simulink model "rlAutoParkingValet3D"  (R2024b)
settings: Solver=VariableStepAuto  StartTime=0.0  StopTime=inf  RelTol=1e-3  AbsTol=1e-4
InitFcn:
  | if ~doTraining
  |     setupActorVehicles(mdl,freeSpotIndex);
  | end
  | egoTargetPose = parkingLot.findGoalPose(vehiclePose,freeSpotIndex,searchDist);
StartFcn:
  | if exist("visualizer","var") && ~doTraining
  |     visualizer.resetVehicle(egoInitialPose,freeSpotIndex,doTraining);
  | end
model workspace: external: MAT-File (data not in the file)
values from neighbouring files (symbols this model uses):
  centerToRear = 1.343    [autoParkingValetParams3D.m]
  doTraining = false    [RL_Parking_And_Control.m]    (also in analisis.m; lanzarSimParalelas.m)
  egoInitialPose = [40 -55 pi/2]    [RL_Parking_And_Control.m]    (also in lanzarSimParalelas.m)
  freeSpotIndex = spotsToSimulate(i)    [RL_Parking_And_Control.m]    (also in analisis.m = 18; autoParkingValetResetFcn3D.m = 21; lanzarSimParalelas.m = 18)
  info = ParkingLotManager.getInfo()    [ParkingLotManager.m]    (also in ParkingLotVisualizer.m = this.Info; RL_Parking_And_Control.m = parkingLot.getInfo(); analisis.m = parkingLot.getInfo(); autoParkingValetResetFcn3D.m)
  K_lqr = dlqr(Ad, Bd, Q, R)    [createLQRForParking3D.m]
  maxLidarDist = 20    [autoParkingValetParams3D.m]
  parkingLot = obj.ParkingLot    [ModeSelector.m]    (also in RL_Parking_And_Control.m = ParkingLotManager; analisis.m = ParkingLotManager; lanzarSimParalelas.m = ParkingLotManager)
  pTracking = 10    [createMPCForParking3D.m]    (also in createNonLinearMPCForParking3D.m)
  searchDist = 10    [RL_Parking_And_Control.m]    (also in analisis.m; lanzarSimParalelas.m)
  speedMax = 2    [autoParkingValetParams3D.m]
  steerMax = pi/4    (= 0.785398163397)    [autoParkingValetParams3D.m]
  terrTol = deg2rad(10)    [autoParkingValetParams3D.m]
  Tf = 50    [RL_Parking_And_Control.m]    (also in analisis.m; lanzarSimParalelas.m)
  trainXBounds = info.TrainingZoneXLimits    [autoParkingValetParams3D.m]    (also in autoParkingValetResetFcn3D.m = [(info.SpotLocations(freeSpotIndex,1) - 6.8125)             )
  trainYBounds = info.TrainingZoneYLimits    [autoParkingValetParams3D.m]    (also in autoParkingValetResetFcn3D.m = [(info.SpotLocations(freeSpotIndex,2) - 9.56)              ()
  Ts = 0.1    [RL_Parking_And_Control.m]    (also in analisis.m; createMPCForParking3D.m; lanzarSimParalelas.m)
  vehiclePose = [10 -32.5 pi]    [RL_Parking_And_Control.m]    (also in analisis.m; lanzarSimParalelas.m)
  xBounds = info.XLimits    [autoParkingValetParams3D.m]
  Xref = [xRef(1:p,:);repmat(xRef(end,:),Tsteps-p,1)]    [ParkingLotManager.m]    (also in createLQRForParking3D.m = parkingLot.createReferenceTrajectory(Ts, Tf); createMPCForParking3D.m = ParkingLotManager.createReferenceTrajectory(Ts,Tf); createNonLinearMPCForParking3D.m = ParkingLotManager.createReferenceTrajectory(Ts,Tf))
  xyerrTol = 0.75    [autoParkingValetParams3D.m]
  yBounds = info.YLimits    [autoParkingValetParams3D.m]
undefined symbols (not defined in the file or in its folder): Sim3dSensor
libraries: sim3dautolib x23, simulink_extras x23, mpclib x2, rllib x1, robotmobilelib x1, sim3dphyssensorlib x1, sim3dlib x1
(part 1 of 2)
settings Model: PauseTimes=24.5  PacingRate=0.089000  Creator=The MathWorks, Inc.  LastModifiedBy=josea
settings SolverCC: AutoScaleAbsTol=off  AlgebraicLoopSolver=TrustRegion  MinimalZcImpactIntegration=on  MaxZcPerStep=1
settings DataIOCC: SaveOutput=off  DSMLogging=off  SaveTime=off
settings DebuggingCC: UnconnectedInputMsg=warning  UnconnectedOutputMsg=warning  UnconnectedLineMsg=warning
settings ModelReferenceCC: EnableRefExpFcnMdlSchedulingChecks=on
settings RTWCC: GPUComputeCapability=3.5  DLArmComputeVersion=19.05

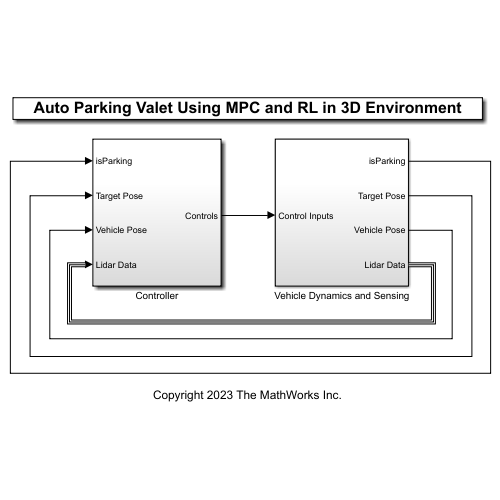
[thumbnail: Simulink's stored preview of the top-level diagram]
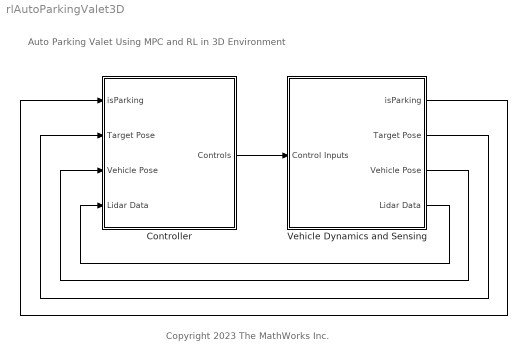
== system rlAutoParkingValet3D ==
  note: Copyright 2023 The MathWorks Inc.
  note: Auto Parking Valet Using MPC and RL in 3D Environment
  Controller : Subsystem
  Vehicle Dynamics and Sensing : Subsystem
  wires:
  Controller/1(Controls) -> Vehicle Dynamics and Sensing/1(Control Inputs)
  Vehicle Dynamics and Sensing/1(isParking) -> Controller/1(isParking)
  Vehicle Dynamics and Sensing/2(Target Pose) -> Controller/2(Target Pose)
  Vehicle Dynamics and Sensing/3(Vehicle Pose) -> Controller/3(Vehicle Pose)
  Vehicle Dynamics and Sensing/4(Lidar Data) -> Controller/4(Lidar Data)

== system rlAutoParkingValet3D/Controller ==
  isParking : Inport
  Target Pose : Inport  Port=2
  Vehicle Pose : Inport  Port=3
  Lidar Data : Inport  Port=4
  MPC Tracking Controller : Subsystem
  Merge : Merge
  NOT : Logic  Operator=NOT  AllPortsSameDT=off  OutDataTypeStr=boolean
  RL Controller : Subsystem
  Controls : Outport
  wires:
  Merge/1 -> Controls/1
  Vehicle Pose/1 -> RL Controller/2(Vehicle Pose), MPC Tracking Controller/1(States)
  Target Pose/1 -> RL Controller/1(Target Pose)
  Lidar Data/1 -> RL Controller/3(Lidar Data)
  RL Controller/1(Controls) -> Merge/2
  MPC Tracking Controller/1(Controls) -> Merge/1
  isParking/1 -> NOT/1, RL Controller/Enable
  NOT/1 -> MPC Tracking Controller/Enable

== system rlAutoParkingValet3D/Vehicle Dynamics and Sensing ==
  Control Inputs : Inport
  Demux : Demux  Outputs=2
  Ego Vehicle Model : Subsystem
  Unreal Engine Visualization and Sensing : Subsystem  InitFcn=|  VariantControl=UnrealOn  mask{EnableUEViz=on, EnablePCViz=on}
      | enableUEViz = get_param(gcb,'enableUEViz');
      | enablePCPlayer = get_param(gcb,'enablePCViz');
      | sim3DConfigBlock = strcat(gcb, "/Simulation 3D Scene Configuration");
      | pcViewerBlock = strcat(gcb, "/Point Cloud Viewer");
      | 
      | if strcmp(enableUEViz, "on")
      |     set_param(sim3DConfigBlock, "EnableWindow", "on");
      | elseif strcmp(enableUEViz, "off")
      |     set_param(sim3DConfigBlock, "EnableWindow", "off");
      | end
      | 
      | if strcmp(enablePCPlayer, "on")
      |     set_param(pcViewerBlock, "OpenAtMdlStart", "on");
      | elseif strcmp(enablePCPlayer, "off")
      |     set_param(pcViewerBlock, "OpenAtMdlStart", "off");
      | end
      mask prompts: EnableUEViz "Enable Unreal Engine visualization"; EnablePCViz "Enable point cloud visualization"
      mask init:
      | enableUEViz = EnableUEViz;
      | enablePCViz = EnablePCViz;
  Vehicle Mode Selector : Subsystem
  isParking : Outport
  Target Pose : Outport  Port=2
  Vehicle Pose : Outport  Port=3
  Lidar Data : Outport  Port=4
  wires:
  Ego Vehicle Model/1(Vehicle Pose (Centroid)) -> Unreal Engine Visualization and Sensing/2(Vehicle Pose (Center)), Vehicle Mode Selector/1(Vehicle Pose)
  Demux/2 -> Unreal Engine Visualization and Sensing/4(Steer Angle), Ego Vehicle Model/2(Steering (rad))  "steering"
  Demux/1 -> Ego Vehicle Model/1(Speed (m/s))
  Unreal Engine Visualization and Sensing/1(Lidar Data) -> Lidar Data/1
  Control Inputs/1 -> Demux/1
  Vehicle Mode Selector/2(isParking) -> isParking/1, Unreal Engine Visualization and Sensing/1(isParking)  "isParking"
  Vehicle Mode Selector/1(TargetPose) -> Target Pose/1
  Ego Vehicle Model/2(Vehicle Pose (Rear Axle)) -> Vehicle Pose/1, Unreal Engine Visualization and Sensing/3(Vehicle Pose (Rear Axle))  "egoPose"

== system rlAutoParkingValet3D/Controller/MPC Tracking Controller ==
  States : Inport
  Enable : EnablePort  StatesWhenEnabling=reset
  Variant Subsystem : Subsystem  Variant=on  VariantControlMode=label  LabelModeActiveChoice=Choice_3  mask{choice=Pure Pursuit}
      mask init:
      | choice = get_param(gcb,'choice');
      | vssBlk = gcb;
      | oldVariant = get_param(gcb,'LabelModeActiveChoice');
      | if strcmp(choice,'Adaptive MPC')
      |     
      |     set_param(vssBlk, 'LabelModeActiveChoice', 'Choice_1');
      | elseif strcmp(choice,'LQR')
      |     
      |     set_param(vssBlk, 'LabelModeActiveChoice', 'Choice_2');
      | elseif strcmp(choice,'Pure Pursuit')
      |     
      |     set_param(vssBlk, 'LabelModeActiveChoice', 'Choice_3');
      | elseif strcmp(choice,'Stanley')
      |     
      |     set_param(vssBlk, 'LabelModeActiveChoice', 'Choice_4');
      | elseif strcmp(choice,'Nonlinear MPC')
      |     
      |     set_param(vssBlk, 'LabelModeActiveChoice', 'Choice_5');
      | end
      mask TypeOptions choice: Adaptive MPC | LQR | Pure Pursuit | Stanley | Nonlinear MPC
  Controls : Outport
  wires:
  States/1 -> Variant Subsystem/1(states)
  Variant Subsystem/1(controls) -> Controls/1

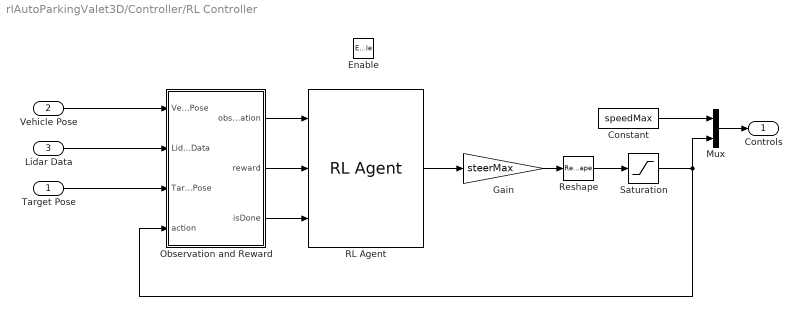
== system rlAutoParkingValet3D/Controller/RL Controller ==
  Target Pose : Inport
  Vehicle Pose : Inport  Port=2
  Lidar Data : Inport  Port=3
  Enable : EnablePort  StatesWhenEnabling=reset
  Constant : Constant  Value=speedMax
  Gain : Gain  Gain=steerMax
  Mux : Mux  Inputs=2
  Observation and Reward : Subsystem
  RL Agent : rllib/RL Agent  Agent=agent  ExternalActionAsInput=off  ProvideLastAction=off  ProvideCumRwd=off  TreatAsDirectFeedthrough=on  UseStrictObservationDataTypes=off
  Reshape : Reshape
  Saturation : Saturate  UpperLimit=steerMax  LowerLimit=-steerMax
  Controls : Outport
  wires:
  Observation and Reward/1(observation) -> RL Agent/1
  Observation and Reward/2(reward) -> RL Agent/2
  Vehicle Pose/1 -> Observation and Reward/1(Vehicle Pose)
  Target Pose/1 -> Observation and Reward/3(Target Pose)
  RL Agent/1 -> Gain/1
  Saturation/1 -> Mux/2, Observation and Reward/4(action)
  Reshape/1 -> Saturation/1
  Constant/1 -> Mux/1
  Mux/1 -> Controls/1
  Gain/1 -> Reshape/1
  Observation and Reward/3(isDone) -> RL Agent/3
  Lidar Data/1 -> Observation and Reward/2(Lidar Data)

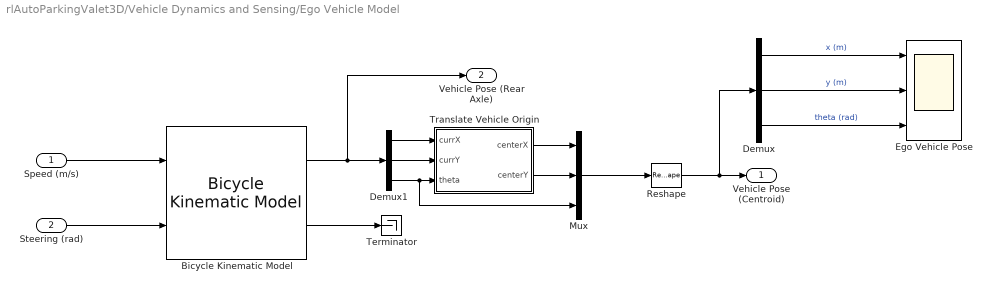
== system rlAutoParkingValet3D/Vehicle Dynamics and Sensing/Ego Vehicle Model ==
  Speed (m/s) : Inport
  Steering (rad) : Inport  Port=2
  Bicycle Kinematic Model : robotmobilelib/Bicycle Kinematic Model  VehicleInputs=Vehicle Speed & Steering Angle  WheelBase=info.CenterToRearDist+info.CenterToFrontDist  VehicleSpeedRange=[-5, 5]  MaxSteeringAngle=steerMax  InitialState=egoInitialPose  SimulateUsing=Interpreted execution
  Demux : Demux  Outputs=3
  Demux1 : Demux  Outputs=3
  Ego Vehicle Pose : Scope  NumInputPorts=3
  Mux : Mux  Inputs=3
  Reshape : Reshape
  Terminator : Terminator
  Translate Vehicle Origin : Subsystem
  Vehicle Pose (Centroid) : Outport
  Vehicle Pose (Rear Axle) : Outport  Port=2
  wires:
  Demux/3 -> Ego Vehicle Pose/3  "theta (rad)"
  Demux/1 -> Ego Vehicle Pose/1  "x (m)"
  Demux/2 -> Ego Vehicle Pose/2  "y (m)"
  Speed (m/s)/1 -> Bicycle Kinematic Model/1
  Steering (rad)/1 -> Bicycle Kinematic Model/2
  Mux/1 -> Reshape/1
  Bicycle Kinematic Model/2 -> Terminator/1
  Bicycle Kinematic Model/1 -> Demux1/1, Vehicle Pose (Rear Axle)/1
  Reshape/1 -> Demux/1, Vehicle Pose (Centroid)/1
  Translate Vehicle Origin/2(centerY) -> Mux/2
  Demux1/1 -> Translate Vehicle Origin/1(currX)
  Demux1/3 -> Mux/3, Translate Vehicle Origin/3(theta)
  Translate Vehicle Origin/1(centerX) -> Mux/1
  Demux1/2 -> Translate Vehicle Origin/2(currY)

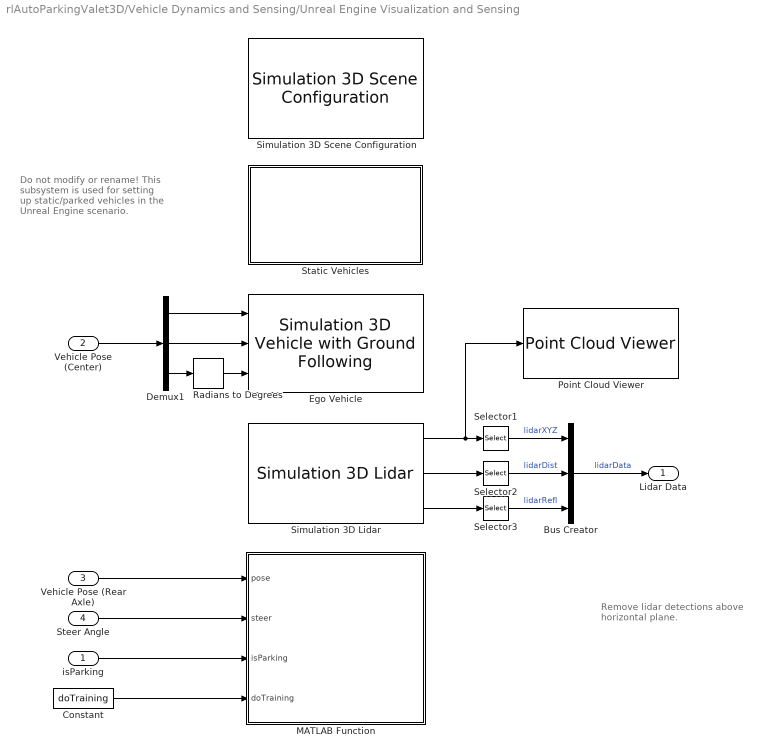
== system rlAutoParkingValet3D/Vehicle Dynamics and Sensing/Unreal Engine Visualization and Sensing ==
  note: Remove lidar detections above horizontal plane.
  note: Do not modify or rename!
      |
      | This subsystem is used for setting up static/parked vehicles in the Unreal Engine scenario.
  isParking : Inport
  Vehicle Pose (Center) : Inport  Port=2
  Vehicle Pose (Rear Axle) : Inport  Port=3
  Steer Angle : Inport  Port=4
  Bus Creator : BusCreator  Inputs=3
  Constant : Constant  Value=doTraining
  Demux1 : Demux  Outputs=3
  Ego Vehicle : sim3dautolib/Simulation 3D Vehicle with Ground Following  Priority=-1  PassVehMesh=Hatchback  MeshPath=/MathWorksSimulation/Vehicles/Muscle/Meshes/SK_MuscleCar.SK_MuscleCar  TrackWidth=1.9  WheelBase=3  WheelRadius=0.35  VehColor=Red  InitialPos=[egoInitialPose(1)+cos(egoInitialPose(3))*centerToRear, egoInitialPose(2)+sin(egoInitialPose(3))*centerToRear, 0]  InitialRot=[0, 0, rad2deg(egoInitialPose(3))]  ActorName=EgoVehicle  SampleTime=-1  ActorType=SimulinkVehicle  ID=C  aMode=3  ActorTag=EgoVehicle  CoordinateScheme=ISO  VehLightsControl=off  HeadlightColor=[ 1, 1, 1 ]  HighBeamIntensity=100000  LowBeamIntensity=60000  HighBeamConeAngle=70  LowBeamConeAngle=70  LeftHeadlightOrientation=[ 0, 0 ]  RightHeadlightOrientation=[ 0, 0 ]  BrakelightIntensity=500  ReverselightIntensity=500  SignallightIntensity=500  SignallightPeriod=1  SignalPulseWidth=50  TransformOutportEnabled=off
      settings: LibrarySourceBlock=drivingsim3d/Simulation 3D Vehicle with Ground Following
  MATLAB Function : MATLAB Function  TreatAsAtomicUnit=on
  Point Cloud Viewer : PointCloudViewer  FigPos=[857.8 630 539.2 508.8]
  Radians to Degrees : simulink_extras/Transformations/Radians to Degrees
  Selector1 : Selector  NumberOfDimensions=3  InputPortWidth=3  IndexOptions=Index vector (dialog),Select all,Select all  Indices=45:60,1,1  OutputSizes=1,1,1
  Selector2 : Selector  NumberOfDimensions=2  InputPortWidth=3  IndexOptions=Index vector (dialog),Select all  Indices=45:60,1  OutputSizes=1,1
  Selector3 : Selector  NumberOfDimensions=2  InputPortWidth=3  IndexOptions=Index vector (dialog),Select all  Indices=45:60,1  OutputSizes=1,1
  Simulation 3D Lidar : sim3dphyssensorlib/Simulation 3D Lidar  Priority=1  sensorTag=Sim3dSensor�  sensorId=2  sensorName=Sim3dSensor�  vehTagList={'EgoVehicle';'Scene Origin';'Vehicle1';'Vehicle10';'Vehicle11';'Vehicle12';'Vehicle13';'Vehicle14';'Vehicle15';'Vehicle16';'Vehicle17';'Vehicle18';'Vehicle19';'Vehicle2';'Vehicle20';'Vehicle21';'Vehicle22';'Vehicle23';'Vehicle3';'Vehicle4';'Vehicle5';'Vehicle6';'Vehicle7';'Vehicle9'}  vehTag=EgoVehicle  mountLoc=Roof center  offsetFlag=on  tmountOffset=[0, 0, 0.2]  rmountOffset=[0, 0, 0]  DetectionRange=maxLidarDist  RangeResolution=0.002  VerticalFOV=lidarVerticalFOV  VerticalResolution=lidarVerticalRes  HorizontalFOV=lidarHorizontalFOV  HorizontalResolution=lidarHorizontalRes  DistanceOutportEnabled=on  ReflectivityOutportEnabled=on  SemanticOutportEnabled=off  TransformOutportEnabled=off  SampleTime=-1  mountPoint=[0 0 1.76]  mountOrientation=[0 0 0]  aMode=3  ID=2
      settings: LibrarySourceBlock=drivingsim3d/Simulation 3D Lidar
  Simulation 3D Scene Configuration : sim3dlib/Simulation 3D Scene Configuration  Priority=0  ProjectFormat=Default Scenes  SceneDesc=Large parking lot  ProjectName=C:\Program Files\MATLAB\R2024b\toolbox\shared\sim3d_projects\automotive_project_windows\UE\WindowsNoEditor\VehicleSimulation.exe  ScenePath=/Game/Maps/HwStrght  EnableOpenDRIVE=off  vehTagList={'Custom';'EgoVehicle';'Scene Origin';'Vehicle1';'Vehicle10';'Vehicle11';'Vehicle12';'Vehicle13';'Vehicle14';'Vehicle15';'Vehicle16';'Vehicle17';'Vehicle18';'Vehicle19';'Vehicle2';'Vehicle20';'Vehicle21';'Vehicle22';'Vehicle23';'Vehicle3';'Vehicle4';'Vehicle5';'Vehicle6';'Vehicle7';'Vehicle9'}  vehTag=EgoVehicle  FreeCameraInitialTranslation=[0, 0, 0]  FreeCameraDefaultInitialTranslation=[-6, 0, 2]  FreeCameraInitialRotation=[0, 0, 0]  FreeCameraDefaultInitialRotation=[0, -15, 0]  OpVisEn=off  Ts=Ts  EnableWindow=on  EnableRemoteAccess=off  EnableWeather=off  SunAzimuth=90  SunAltitude=40.0  EnableGeospatialSun=off  Latitude=0  Longitude=0  Date=2023-01-01  Time=10:30:00  GeoTimeZone=-5.0  SunDaylightSaving=off  wind=1  clouds=10  EnableVolumetricClouds=off  CloudCoverage=0  CloudAltitude=6  fog=0  rain=0  RaindropsEffect=off  SnowDensity=0  EnableGeospatial=off  UseTrueOrigin=off  OriginHeight=200  OriginLatitude=40.744652  OriginLongitude=-73.988864  MapStyle=Aerial  AdditionalAssetIDs=[]  UseAdvancedSunSky=off  SolarTime=11  TimeZone=-5  Day=21  Month=9  Year=2022  UseDaylightSavingTime=on  DSTStartDay=10  DSTStartMonth=3  DSTEndDay=3  DSTEndMonth=11  DSTSwitchHour=2  sensorTag=MainCamera2  sensorId=2  sensorName=MainCamera2  mountLoc=Origin  offsetFlag=off  tmountOffset=[0, 0, 0]  rmountOffset=[0, 0, 0]  HorizontalResolution=1280  VerticalResolution=720  HorizontalFOV=60  mountPoint=[0 0 0]  mountOrientation=[0 0 0]  aMode=3  ID=2  GeoTrigger=Inactive
      settings: LibrarySourceBlock=drivingsim3d/Simulation 3D Scene Configuration
  Static Vehicles : Subsystem  Priority=-1
  Lidar Data : Outport
  wires:
  Vehicle Pose (Center)/1 -> Demux1/1
  Radians to Degrees/1 -> Ego Vehicle/3
  Demux1/1 -> Ego Vehicle/1
  Demux1/2 -> Ego Vehicle/2
  Demux1/3 -> Radians to Degrees/1
  Simulation 3D Lidar/1 -> Point Cloud Viewer/1, Selector1/1
  Simulation 3D Lidar/2 -> Selector2/1
  Simulation 3D Lidar/3 -> Selector3/1
  Bus Creator/1 -> Lidar Data/1  "lidarData"
  Selector1/1 -> Bus Creator/1  "lidarXYZ"
  Selector2/1 -> Bus Creator/2  "lidarDist"
  Selector3/1 -> Bus Creator/3  "lidarRefl"
  Steer Angle/1 -> MATLAB Function/2(steer)
  isParking/1 -> MATLAB Function/3(isParking)
  Constant/1 -> MATLAB Function/4(doTraining)
  Vehicle Pose (Rear Axle)/1 -> MATLAB Function/1(pose)

== system rlAutoParkingValet3D/Vehicle Dynamics and Sensing/Vehicle Mode Selector ==
  Vehicle Pose : Inport
  Constant : Constant  Value=doTraining
  Constant1 : Constant  Value=egoTargetPose
  Hold : Subsystem
  Mode Selector : MATLABSystem  System=ModeSelector  MaxDepth=searchDist  MaxViewAngle=2*pi/3  FreeSpotIndex=freeSpotIndex  ParkingLot=parkingLot
      mask Type: ModeSelector
      mask Display:
      | disp(['Mode' char(10) 'Selector']);
      | port_label('input',1,'Ego Pose');
      | port_label('output',1,'Spot Found');
      | port_label('output',2,'Target Spot Pose');
  OR : Logic  Operator=OR  AllPortsSameDT=off  OutDataTypeStr=boolean
  Switch : Switch  Threshold=1  SaturateOnIntegerOverflow=off  InputSameDT=off
  TargetPose : Outport
  isParking : Outport  Port=2
  wires:
  Hold/1(y) -> isParking/1
  Switch/1 -> TargetPose/1
  Vehicle Pose/1 -> Mode Selector/1
  Mode Selector/2 -> Switch/3
  Constant/1 -> Switch/2, OR/2
  Constant1/1 -> Switch/1
  OR/1 -> Hold/1(u)
  Mode Selector/1 -> OR/1

== system rlAutoParkingValet3D/Controller/MPC Tracking Controller/Variant Subsystem ==
  note: 1) Add Subsystem or Model blocks as valid variant choices.
      | 2) You cannot connect blocks at this level. At simulation, connectivity is automatically
      | determined, based on the active variant and port name matching.
  states : Inport
  Adaptive MPC : Subsystem  VariantControl=Choice_1
  LQR : Subsystem  VariantControl=Choice_2
  Nonlinear MPC : Subsystem  VariantControl=Choice_5
  Pure Pursuit : Subsystem  VariantControl=Choice_3
  Stanley : Subsystem  VariantControl=Choice_4
  controls : Outport

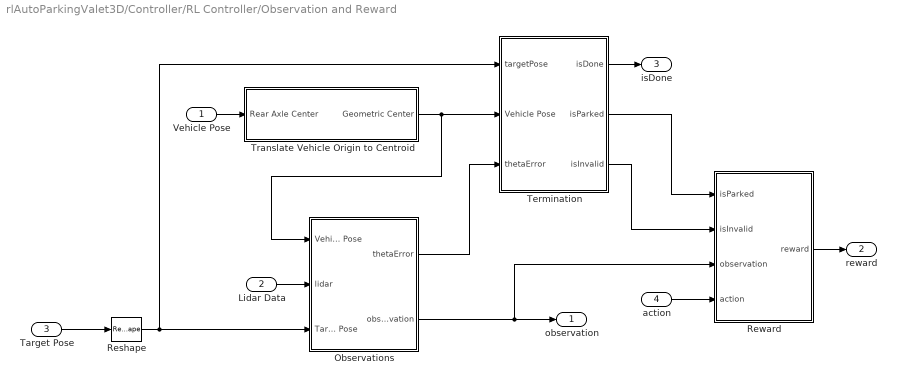
== system rlAutoParkingValet3D/Controller/RL Controller/Observation and Reward ==
  Vehicle Pose : Inport
  Lidar Data : Inport  Port=2
  Target Pose : Inport  Port=3
  action : Inport  Port=4
  Observations : Subsystem
  Reshape : Reshape
  Reward : Subsystem
  Termination : Subsystem
  Translate Vehicle Origin to Centroid : Subsystem
  observation : Outport
  reward : Outport  Port=2
  isDone : Outport  Port=3
  wires:
  action/1 -> Reward/4(action)
  Reward/1(reward) -> reward/1
  Target Pose/1 -> Reshape/1
  Observations/2(observation) -> observation/1, Reward/3(observation)
  Lidar Data/1 -> Observations/2(lidar)
  Termination/2(isParked) -> Reward/1(isParked)
  Reshape/1 -> Observations/3(Target Pose), Termination/1(targetPose)
  Termination/1(isDone) -> isDone/1
  Termination/3(isInvalid) -> Reward/2(isInvalid)
  Translate Vehicle Origin to Centroid/1(Geometric Center) -> Observations/1(Vehicle Pose), Termination/2(Vehicle Pose)
  Vehicle Pose/1 -> Translate Vehicle Origin to Centroid/1(Rear Axle Center)
  Observations/1(thetaError) -> Termination/3(thetaError)

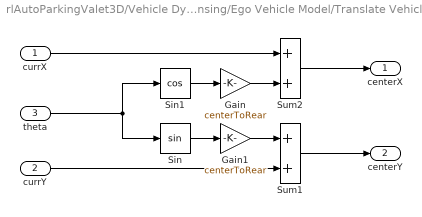
== system rlAutoParkingValet3D/Vehicle Dynamics and Sensing/Ego Vehicle Model/Translate Vehicle Origin ==
  currX : Inport
  currY : Inport  Port=2
  theta : Inport  Port=3
  Gain : Gain  Gain=centerToRear
  Gain1 : Gain  Gain=centerToRear
  Sin : Trigonometry
  Sin1 : Trigonometry  Operator=cos
  Sum1 : Sum
  Sum2 : Sum
  centerX : Outport
  centerY : Outport  Port=2
  wires:
  Sum1/1 -> centerY/1
  currY/1 -> Sum1/2
  theta/1 -> Sin/1, Sin1/1
  Sin/1 -> Gain1/1
  Sin1/1 -> Gain/1
  currX/1 -> Sum2/1
  Sum2/1 -> centerX/1
  Gain/1 -> Sum2/2
  Gain1/1 -> Sum1/1

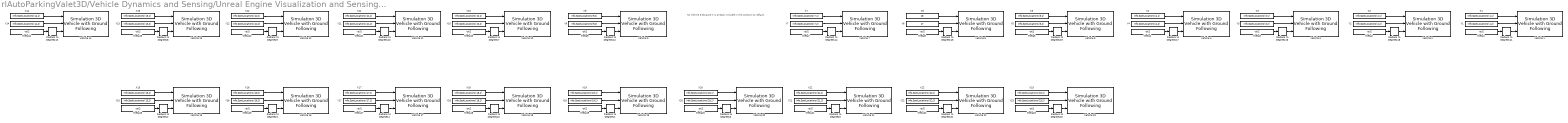
== system rlAutoParkingValet3D/Vehicle Dynamics and Sensing/Unreal Engine Visualization and Sensing/Static Vehicles ==
  note: No Vehicle 8 because it is already included in the scenario by default.
  Radians to Degrees{1..22} (22 alike) : simulink_extras/Transformations/Radians to Degrees
  Vehicle 1 : sim3dautolib/Simulation 3D Vehicle with Ground Following  Priority=-1  PassVehMesh=Sedan  MeshPath=/MathWorksAutomotiveContent/Vehicles/Muscle/Meshes/SK_MuscleCar.SK_MuscleCar  TrackWidth=1.9  WheelBase=3  WheelRadius=0.35  VehColor=White  InitialPos=[info.SpotLocations(1,1), info.SpotLocations(1,2), 0]  InitialRot=[0 0 -pi/2]  ActorName=Vehicle1  SampleTime=Ts  ActorType=SimulinkVehicle  ID=C  aMode=3  ActorTag=Vehicle1  CoordinateScheme=ISO  VehLightsControl=off  HeadlightColor=[ 1, 1, 1 ]  HighBeamIntensity=100000  LowBeamIntensity=60000  HighBeamConeAngle=70  LowBeamConeAngle=70  LeftHeadlightOrientation=[ 0, 0 ]  RightHeadlightOrientation=[ 0, 0 ]  BrakelightIntensity=500  ReverselightIntensity=500  SignallightIntensity=500  SignallightPeriod=1  SignalPulseWidth=50  TransformOutportEnabled=off
      settings: LibrarySourceBlock=drivingsim3d/Simulation 3D Vehicle with Ground Following
  Vehicle 10 : sim3dautolib/Simulation 3D Vehicle with Ground Following  Priority=-1  PassVehMesh=Sedan  MeshPath=/MathWorksAutomotiveContent/Vehicles/Muscle/Meshes/SK_MuscleCar.SK_MuscleCar  TrackWidth=1.9  WheelBase=3  WheelRadius=0.35  VehColor=Red  InitialPos=[info.SpotLocations(10,1), info.SpotLocations(10,2), 0]  InitialRot=[0 0 -pi/2]  ActorName=Vehicle10  SampleTime=Ts  ActorType=SimulinkVehicle  ID=C  aMode=3  ActorTag=Vehicle10  CoordinateScheme=ISO  VehLightsControl=off  HeadlightColor=[ 1, 1, 1 ]  HighBeamIntensity=100000  LowBeamIntensity=60000  HighBeamConeAngle=70  LowBeamConeAngle=70  LeftHeadlightOrientation=[ 0, 0 ]  RightHeadlightOrientation=[ 0, 0 ]  BrakelightIntensity=500  ReverselightIntensity=500  SignallightIntensity=500  SignallightPeriod=1  SignalPulseWidth=50  TransformOutportEnabled=off
      settings: LibrarySourceBlock=drivingsim3d/Simulation 3D Vehicle with Ground Following
  Vehicle 11 : sim3dautolib/Simulation 3D Vehicle with Ground Following  Priority=-1  PassVehMesh=Muscle car  MeshPath=/MathWorksAutomotiveContent/Vehicles/Muscle/Meshes/SK_MuscleCar.SK_MuscleCar  TrackWidth=1.9  WheelBase=3  WheelRadius=0.35  VehColor=Black  InitialPos=[info.SpotLocations(11,1), info.SpotLocations(11,2), 0]  InitialRot=[0 0 -pi/2]  ActorName=Vehicle11  SampleTime=Ts  ActorType=SimulinkVehicle  ID=C  aMode=3  ActorTag=Vehicle11  CoordinateScheme=ISO  VehLightsControl=off  HeadlightColor=[ 1, 1, 1 ]  HighBeamIntensity=100000  LowBeamIntensity=60000  HighBeamConeAngle=70  LowBeamConeAngle=70  LeftHeadlightOrientation=[ 0, 0 ]  RightHeadlightOrientation=[ 0, 0 ]  BrakelightIntensity=500  ReverselightIntensity=500  SignallightIntensity=500  SignallightPeriod=1  SignalPulseWidth=50  TransformOutportEnabled=off
      settings: LibrarySourceBlock=drivingsim3d/Simulation 3D Vehicle with Ground Following
  Vehicle 12 : sim3dautolib/Simulation 3D Vehicle with Ground Following  Priority=-1  PassVehMesh=Sport utility vehicle  MeshPath=/MathWorksAutomotiveContent/Vehicles/Muscle/Meshes/SK_MuscleCar.SK_MuscleCar  TrackWidth=1.9  WheelBase=3  WheelRadius=0.35  VehColor=White  InitialPos=[info.SpotLocations(12,1), info.SpotLocations(12,2), 0]  InitialRot=[0 0 -pi/2]  ActorName=Vehicle12  SampleTime=Ts  ActorType=SimulinkVehicle  ID=C  aMode=3  ActorTag=Vehicle12  CoordinateScheme=ISO  VehLightsControl=off  HeadlightColor=[ 1, 1, 1 ]  HighBeamIntensity=100000  LowBeamIntensity=60000  HighBeamConeAngle=70  LowBeamConeAngle=70  LeftHeadlightOrientation=[ 0, 0 ]  RightHeadlightOrientation=[ 0, 0 ]  BrakelightIntensity=500  ReverselightIntensity=500  SignallightIntensity=500  SignallightPeriod=1  SignalPulseWidth=50  TransformOutportEnabled=off
      settings: LibrarySourceBlock=drivingsim3d/Simulation 3D Vehicle with Ground Following
  Vehicle 13 : sim3dautolib/Simulation 3D Vehicle with Ground Following  Priority=-1  PassVehMesh=Sedan  MeshPath=/MathWorksAutomotiveContent/Vehicles/Muscle/Meshes/SK_MuscleCar.SK_MuscleCar  TrackWidth=1.9  WheelBase=3  WheelRadius=0.35  VehColor=Blue  InitialPos=[info.SpotLocations(13,1), info.SpotLocations(13,2), 0]  InitialRot=[0 0 -pi/2]  ActorName=Vehicle13  SampleTime=Ts  ActorType=SimulinkVehicle  ID=C  aMode=3  ActorTag=Vehicle13  CoordinateScheme=ISO  VehLightsControl=off  HeadlightColor=[ 1, 1, 1 ]  HighBeamIntensity=100000  LowBeamIntensity=60000  HighBeamConeAngle=70  LowBeamConeAngle=70  LeftHeadlightOrientation=[ 0, 0 ]  RightHeadlightOrientation=[ 0, 0 ]  BrakelightIntensity=500  ReverselightIntensity=500  SignallightIntensity=500  SignallightPeriod=1  SignalPulseWidth=50  TransformOutportEnabled=off
      settings: LibrarySourceBlock=drivingsim3d/Simulation 3D Vehicle with Ground Following
  Vehicle 14 : sim3dautolib/Simulation 3D Vehicle with Ground Following  Priority=-1  PassVehMesh=Sedan  MeshPath=/MathWorksAutomotiveContent/Vehicles/Muscle/Meshes/SK_MuscleCar.SK_MuscleCar  TrackWidth=1.9  WheelBase=3  WheelRadius=0.35  VehColor=Blue  InitialPos=[info.SpotLocations(14,1), info.SpotLocations(14,2), 0]  InitialRot=[0 0 -pi/2]  ActorName=Vehicle14  SampleTime=Ts  ActorType=SimulinkVehicle  ID=C  aMode=3  ActorTag=Vehicle14  CoordinateScheme=ISO  VehLightsControl=off  HeadlightColor=[ 1, 1, 1 ]  HighBeamIntensity=100000  LowBeamIntensity=60000  HighBeamConeAngle=70  LowBeamConeAngle=70  LeftHeadlightOrientation=[ 0, 0 ]  RightHeadlightOrientation=[ 0, 0 ]  BrakelightIntensity=500  ReverselightIntensity=500  SignallightIntensity=500  SignallightPeriod=1  SignalPulseWidth=50  TransformOutportEnabled=off
      settings: LibrarySourceBlock=drivingsim3d/Simulation 3D Vehicle with Ground Following
  Vehicle 15 : sim3dautolib/Simulation 3D Vehicle with Ground Following  Priority=-1  PassVehMesh=Sedan  MeshPath=/MathWorksAutomotiveContent/Vehicles/Muscle/Meshes/SK_MuscleCar.SK_MuscleCar  TrackWidth=1.9  WheelBase=3  WheelRadius=0.35  VehColor=Blue  InitialPos=[info.SpotLocations(15,1), info.SpotLocations(15,2), 0]  InitialRot=[0 0 -pi/2]  ActorName=Vehicle15  SampleTime=Ts  ActorType=SimulinkVehicle  ID=C  aMode=3  ActorTag=Vehicle15  CoordinateScheme=ISO  VehLightsControl=off  HeadlightColor=[ 1, 1, 1 ]  HighBeamIntensity=100000  LowBeamIntensity=60000  HighBeamConeAngle=70  LowBeamConeAngle=70  LeftHeadlightOrientation=[ 0, 0 ]  RightHeadlightOrientation=[ 0, 0 ]  BrakelightIntensity=500  ReverselightIntensity=500  SignallightIntensity=500  SignallightPeriod=1  SignalPulseWidth=50  TransformOutportEnabled=off
      settings: LibrarySourceBlock=drivingsim3d/Simulation 3D Vehicle with Ground Following
  Vehicle 16 : sim3dautolib/Simulation 3D Vehicle with Ground Following  Priority=-1  PassVehMesh=Sport utility vehicle  MeshPath=/MathWorksAutomotiveContent/Vehicles/Muscle/Meshes/SK_MuscleCar.SK_MuscleCar  TrackWidth=1.9  WheelBase=3  WheelRadius=0.35  VehColor=White  InitialPos=[info.SpotLocations(16,1), info.SpotLocations(16,2), 0]  InitialRot=[0 0 -pi/2]  ActorName=Vehicle16  SampleTime=Ts  ActorType=SimulinkVehicle  ID=C  aMode=3  ActorTag=Vehicle16  CoordinateScheme=ISO  VehLightsControl=off  HeadlightColor=[ 1, 1, 1 ]  HighBeamIntensity=100000  LowBeamIntensity=60000  HighBeamConeAngle=70  LowBeamConeAngle=70  LeftHeadlightOrientation=[ 0, 0 ]  RightHeadlightOrientation=[ 0, 0 ]  BrakelightIntensity=500  ReverselightIntensity=500  SignallightIntensity=500  SignallightPeriod=1  SignalPulseWidth=50  TransformOutportEnabled=off
      settings: LibrarySourceBlock=drivingsim3d/Simulation 3D Vehicle with Ground Following
  Vehicle 17 : sim3dautolib/Simulation 3D Vehicle with Ground Following  Priority=-1  PassVehMesh=Hatchback  MeshPath=/MathWorksAutomotiveContent/Vehicles/Muscle/Meshes/SK_MuscleCar.SK_MuscleCar  TrackWidth=1.9  WheelBase=3  WheelRadius=0.35  VehColor=Blue  InitialPos=[info.SpotLocations(17,1), info.SpotLocations(17,2), 0]  InitialRot=[0 0 -pi/2]  ActorName=Vehicle17  SampleTime=Ts  ActorType=SimulinkVehicle  ID=C  aMode=3  ActorTag=Vehicle17  CoordinateScheme=ISO  VehLightsControl=off  HeadlightColor=[ 1, 1, 1 ]  HighBeamIntensity=100000  LowBeamIntensity=60000  HighBeamConeAngle=70  LowBeamConeAngle=70  LeftHeadlightOrientation=[ 0, 0 ]  RightHeadlightOrientation=[ 0, 0 ]  BrakelightIntensity=500  ReverselightIntensity=500  SignallightIntensity=500  SignallightPeriod=1  SignalPulseWidth=50  TransformOutportEnabled=off
      settings: LibrarySourceBlock=drivingsim3d/Simulation 3D Vehicle with Ground Following
  Vehicle 18 : sim3dautolib/Simulation 3D Vehicle with Ground Following  Priority=-1  PassVehMesh=Sedan  MeshPath=/MathWorksAutomotiveContent/Vehicles/Muscle/Meshes/SK_MuscleCar.SK_MuscleCar  TrackWidth=1.9  WheelBase=3  WheelRadius=0.35  VehColor=Red  InitialPos=[info.SpotLocations(18,1), info.SpotLocations(18,2), 0]  InitialRot=[0 0 -pi/2]  ActorName=Vehicle18  SampleTime=Ts  ActorType=SimulinkVehicle  ID=C  aMode=3  ActorTag=Vehicle18  CoordinateScheme=ISO  VehLightsControl=off  HeadlightColor=[ 1, 1, 1 ]  HighBeamIntensity=100000  LowBeamIntensity=60000  HighBeamConeAngle=70  LowBeamConeAngle=70  LeftHeadlightOrientation=[ 0, 0 ]  RightHeadlightOrientation=[ 0, 0 ]  BrakelightIntensity=500  ReverselightIntensity=500  SignallightIntensity=500  SignallightPeriod=1  SignalPulseWidth=50  TransformOutportEnabled=off
      settings: LibrarySourceBlock=drivingsim3d/Simulation 3D Vehicle with Ground Following
  Vehicle 19 : sim3dautolib/Simulation 3D Vehicle with Ground Following  Priority=-1  PassVehMesh=Sedan  MeshPath=/MathWorksAutomotiveContent/Vehicles/Muscle/Meshes/SK_MuscleCar.SK_MuscleCar  TrackWidth=1.9  WheelBase=3  WheelRadius=0.35  VehColor=Black  InitialPos=[info.SpotLocations(19,1), info.SpotLocations(19,2), 0]  InitialRot=[0 0 -pi/2]  ActorName=Vehicle19  SampleTime=Ts  ActorType=SimulinkVehicle  ID=C  aMode=3  ActorTag=Vehicle19  CoordinateScheme=ISO  VehLightsControl=off  HeadlightColor=[ 1, 1, 1 ]  HighBeamIntensity=100000  LowBeamIntensity=60000  HighBeamConeAngle=70  LowBeamConeAngle=70  LeftHeadlightOrientation=[ 0, 0 ]  RightHeadlightOrientation=[ 0, 0 ]  BrakelightIntensity=500  ReverselightIntensity=500  SignallightIntensity=500  SignallightPeriod=1  SignalPulseWidth=50  TransformOutportEnabled=off
      settings: LibrarySourceBlock=drivingsim3d/Simulation 3D Vehicle with Ground Following
  Vehicle 2 : sim3dautolib/Simulation 3D Vehicle with Ground Following  Priority=-1  PassVehMesh=Small pickup truck  MeshPath=/MathWorksAutomotiveContent/Vehicles/Muscle/Meshes/SK_MuscleCar.SK_MuscleCar  TrackWidth=1.9  WheelBase=3  WheelRadius=0.35  VehColor=Black  InitialPos=[info.SpotLocations(2,1), info.SpotLocations(2,2), 0]  InitialRot=[0 0 -pi/2]  ActorName=Vehicle2  SampleTime=Ts  ActorType=SimulinkVehicle  ID=C  aMode=3  ActorTag=Vehicle2  CoordinateScheme=ISO  VehLightsControl=off  HeadlightColor=[ 1, 1, 1 ]  HighBeamIntensity=100000  LowBeamIntensity=60000  HighBeamConeAngle=70  LowBeamConeAngle=70  LeftHeadlightOrientation=[ 0, 0 ]  RightHeadlightOrientation=[ 0, 0 ]  BrakelightIntensity=500  ReverselightIntensity=500  SignallightIntensity=500  SignallightPeriod=1  SignalPulseWidth=50  TransformOutportEnabled=off
      settings: LibrarySourceBlock=drivingsim3d/Simulation 3D Vehicle with Ground Following
  Vehicle 20 : sim3dautolib/Simulation 3D Vehicle with Ground Following  Priority=-1  PassVehMesh=Sedan  MeshPath=/MathWorksAutomotiveContent/Vehicles/Muscle/Meshes/SK_MuscleCar.SK_MuscleCar  TrackWidth=1.9  WheelBase=3  WheelRadius=0.35  VehColor=Yellow  InitialPos=[info.SpotLocations(20,1), info.SpotLocations(20,2), 0]  InitialRot=[0 0 -pi/2]  ActorName=Vehicle20  SampleTime=Ts  ActorType=SimulinkVehicle  ID=C  aMode=3  ActorTag=Vehicle20  CoordinateScheme=ISO  VehLightsControl=off  HeadlightColor=[ 1, 1, 1 ]  HighBeamIntensity=100000  LowBeamIntensity=60000  HighBeamConeAngle=70  LowBeamConeAngle=70  LeftHeadlightOrientation=[ 0, 0 ]  RightHeadlightOrientation=[ 0, 0 ]  BrakelightIntensity=500  ReverselightIntensity=500  SignallightIntensity=500  SignallightPeriod=1  SignalPulseWidth=50  TransformOutportEnabled=off
      settings: LibrarySourceBlock=drivingsim3d/Simulation 3D Vehicle with Ground Following
  Vehicle 21 : sim3dautolib/Simulation 3D Vehicle with Ground Following  Priority=-1  PassVehMesh=Sport utility vehicle  MeshPath=/MathWorksAutomotiveContent/Vehicles/Muscle/Meshes/SK_MuscleCar.SK_MuscleCar  TrackWidth=1.9  WheelBase=3  WheelRadius=0.35  VehColor=Black  InitialPos=[info.SpotLocations(21,1), info.SpotLocations(21,2), 0]  InitialRot=[0 0 -pi/2]  ActorName=Vehicle21  SampleTime=Ts  ActorType=SimulinkVehicle  ID=C  aMode=3  ActorTag=Vehicle21  CoordinateScheme=ISO  VehLightsControl=off  HeadlightColor=[ 1, 1, 1 ]  HighBeamIntensity=100000  LowBeamIntensity=60000  HighBeamConeAngle=70  LowBeamConeAngle=70  LeftHeadlightOrientation=[ 0, 0 ]  RightHeadlightOrientation=[ 0, 0 ]  BrakelightIntensity=500  ReverselightIntensity=500  SignallightIntensity=500  SignallightPeriod=1  SignalPulseWidth=50  TransformOutportEnabled=off
      settings: LibrarySourceBlock=drivingsim3d/Simulation 3D Vehicle with Ground Following
  Vehicle 22 : sim3dautolib/Simulation 3D Vehicle with Ground Following  Priority=-1  PassVehMesh=Hatchback  MeshPath=/MathWorksAutomotiveContent/Vehicles/Muscle/Meshes/SK_MuscleCar.SK_MuscleCar  TrackWidth=1.9  WheelBase=3  WheelRadius=0.35  VehColor=Red  InitialPos=[info.SpotLocations(22,1), info.SpotLocations(22,2), 0]  InitialRot=[0 0 -pi/2]  ActorName=Vehicle22  SampleTime=Ts  ActorType=SimulinkVehicle  ID=C  aMode=3  ActorTag=Vehicle22  CoordinateScheme=ISO  VehLightsControl=off  HeadlightColor=[ 1, 1, 1 ]  HighBeamIntensity=100000  LowBeamIntensity=60000  HighBeamConeAngle=70  LowBeamConeAngle=70  LeftHeadlightOrientation=[ 0, 0 ]  RightHeadlightOrientation=[ 0, 0 ]  BrakelightIntensity=500  ReverselightIntensity=500  SignallightIntensity=500  SignallightPeriod=1  SignalPulseWidth=50  TransformOutportEnabled=off
      settings: LibrarySourceBlock=drivingsim3d/Simulation 3D Vehicle with Ground Following
  Vehicle 23 : sim3dautolib/Simulation 3D Vehicle with Ground Following  Priority=-1  PassVehMesh=Sport utility vehicle  MeshPath=/MathWorksAutomotiveContent/Vehicles/Muscle/Meshes/SK_MuscleCar.SK_MuscleCar  TrackWidth=1.9  WheelBase=3  WheelRadius=0.35  VehColor=White  InitialPos=[info.SpotLocations(23,1), info.SpotLocations(23,2), 0]  InitialRot=[0 0 -pi/2]  ActorName=Vehicle23  SampleTime=Ts  ActorType=SimulinkVehicle  ID=C  aMode=3  ActorTag=Vehicle23  CoordinateScheme=ISO  VehLightsControl=off  HeadlightColor=[ 1, 1, 1 ]  HighBeamIntensity=100000  LowBeamIntensity=60000  HighBeamConeAngle=70  LowBeamConeAngle=70  LeftHeadlightOrientation=[ 0, 0 ]  RightHeadlightOrientation=[ 0, 0 ]  BrakelightIntensity=500  ReverselightIntensity=500  SignallightIntensity=500  SignallightPeriod=1  SignalPulseWidth=50  TransformOutportEnabled=off
      settings: LibrarySourceBlock=drivingsim3d/Simulation 3D Vehicle with Ground Following
  Vehicle 3 : sim3dautolib/Simulation 3D Vehicle with Ground Following  Priority=-1  PassVehMesh=Sport utility vehicle  MeshPath=/MathWorksAutomotiveContent/Vehicles/Muscle/Meshes/SK_MuscleCar.SK_MuscleCar  TrackWidth=1.9  WheelBase=3  WheelRadius=0.35  VehColor=Red  InitialPos=[info.SpotLocations(3,1), info.SpotLocations(3,2), 0]  InitialRot=[0 0 -pi/2]  ActorName=Vehicle3  SampleTime=Ts  ActorType=SimulinkVehicle  ID=C  aMode=3  ActorTag=Vehicle3  CoordinateScheme=ISO  VehLightsControl=off  HeadlightColor=[ 1, 1, 1 ]  HighBeamIntensity=100000  LowBeamIntensity=60000  HighBeamConeAngle=70  LowBeamConeAngle=70  LeftHeadlightOrientation=[ 0, 0 ]  RightHeadlightOrientation=[ 0, 0 ]  BrakelightIntensity=500  ReverselightIntensity=500  SignallightIntensity=500  SignallightPeriod=1  SignalPulseWidth=50  TransformOutportEnabled=off
      settings: LibrarySourceBlock=drivingsim3d/Simulation 3D Vehicle with Ground Following
  Vehicle 4 : sim3dautolib/Simulation 3D Vehicle with Ground Following  Priority=-1  PassVehMesh=Muscle car  MeshPath=/MathWorksAutomotiveContent/Vehicles/Muscle/Meshes/SK_MuscleCar.SK_MuscleCar  TrackWidth=1.9  WheelBase=3  WheelRadius=0.35  VehColor=White  InitialPos=[info.SpotLocations(4,1), info.SpotLocations(4,2), 0]  InitialRot=[0 0 -pi/2]  ActorName=Vehicle4  SampleTime=Ts  ActorType=SimulinkVehicle  ID=C  aMode=3  ActorTag=Vehicle4  CoordinateScheme=ISO  VehLightsControl=off  HeadlightColor=[ 1, 1, 1 ]  HighBeamIntensity=100000  LowBeamIntensity=60000  HighBeamConeAngle=70  LowBeamConeAngle=70  LeftHeadlightOrientation=[ 0, 0 ]  RightHeadlightOrientation=[ 0, 0 ]  BrakelightIntensity=500  ReverselightIntensity=500  SignallightIntensity=500  SignallightPeriod=1  SignalPulseWidth=50  TransformOutportEnabled=off
      settings: LibrarySourceBlock=drivingsim3d/Simulation 3D Vehicle with Ground Following
  Vehicle 5 : sim3dautolib/Simulation 3D Vehicle with Ground Following  Priority=-1  PassVehMesh=Muscle car  MeshPath=/MathWorksAutomotiveContent/Vehicles/Muscle/Meshes/SK_MuscleCar.SK_MuscleCar  TrackWidth=1.9  WheelBase=3  WheelRadius=0.35  VehColor=Red  InitialPos=[info.SpotLocations(5,1), info.SpotLocations(5,2), 0]  InitialRot=[0 0 -pi/2]  ActorName=Vehicle5  SampleTime=Ts  ActorType=SimulinkVehicle  ID=C  aMode=3  ActorTag=Vehicle5  CoordinateScheme=ISO  VehLightsControl=off  HeadlightColor=[ 1, 1, 1 ]  HighBeamIntensity=100000  LowBeamIntensity=60000  HighBeamConeAngle=70  LowBeamConeAngle=70  LeftHeadlightOrientation=[ 0, 0 ]  RightHeadlightOrientation=[ 0, 0 ]  BrakelightIntensity=500  ReverselightIntensity=500  SignallightIntensity=500  SignallightPeriod=1  SignalPulseWidth=50  TransformOutportEnabled=off
      settings: LibrarySourceBlock=drivingsim3d/Simulation 3D Vehicle with Ground Following
  Vehicle 6 : sim3dautolib/Simulation 3D Vehicle with Ground Following  Priority=-1  PassVehMesh=Sedan  MeshPath=/MathWorksAutomotiveContent/Vehicles/Muscle/Meshes/SK_MuscleCar.SK_MuscleCar  TrackWidth=1.9  WheelBase=3  WheelRadius=0.35  VehColor=Silver  InitialPos=[16, -17, 0]  InitialRot=[0 0 -pi/2]  ActorName=Vehicle6  SampleTime=Ts  ActorType=SimulinkVehicle  ID=C  aMode=3  ActorTag=Vehicle6  CoordinateScheme=ISO  VehLightsControl=off  HeadlightColor=[ 1, 1, 1 ]  HighBeamIntensity=100000  LowBeamIntensity=60000  HighBeamConeAngle=70  LowBeamConeAngle=70  LeftHeadlightOrientation=[ 0, 0 ]  RightHeadlightOrientation=[ 0, 0 ]  BrakelightIntensity=500  ReverselightIntensity=500  SignallightIntensity=500  SignallightPeriod=1  SignalPulseWidth=50  TransformOutportEnabled=off
      settings: LibrarySourceBlock=drivingsim3d/Simulation 3D Vehicle with Ground Following
  Vehicle 7 : sim3dautolib/Simulation 3D Vehicle with Ground Following  Priority=-1  PassVehMesh=Hatchback  MeshPath=/MathWorksAutomotiveContent/Vehicles/Muscle/Meshes/SK_MuscleCar.SK_MuscleCar  TrackWidth=1.9  WheelBase=3  WheelRadius=0.35  VehColor=Black  InitialPos=[info.SpotLocations(7,1), info.SpotLocations(7,2), 0]  InitialRot=[0 0 -pi/2]  ActorName=Vehicle7  SampleTime=Ts  ActorType=SimulinkVehicle  ID=C  aMode=3  ActorTag=Vehicle7  CoordinateScheme=ISO  VehLightsControl=off  HeadlightColor=[ 1, 1, 1 ]  HighBeamIntensity=100000  LowBeamIntensity=60000  HighBeamConeAngle=70  LowBeamConeAngle=70  LeftHeadlightOrientation=[ 0, 0 ]  RightHeadlightOrientation=[ 0, 0 ]  BrakelightIntensity=500  ReverselightIntensity=500  SignallightIntensity=500  SignallightPeriod=1  SignalPulseWidth=50  TransformOutportEnabled=off
      settings: LibrarySourceBlock=drivingsim3d/Simulation 3D Vehicle with Ground Following
  Vehicle 9 : sim3dautolib/Simulation 3D Vehicle with Ground Following  Priority=-1  PassVehMesh=Sedan  MeshPath=/MathWorksAutomotiveContent/Vehicles/Muscle/Meshes/SK_MuscleCar.SK_MuscleCar  TrackWidth=1.9  WheelBase=3  WheelRadius=0.35  VehColor=Silver  InitialPos=[info.SpotLocations(9,1), info.SpotLocations(9,2), 0]  InitialRot=[0 0 -pi/2]  ActorName=Vehicle9  SampleTime=Ts  ActorType=SimulinkVehicle  ID=C  aMode=3  ActorTag=Vehicle9  CoordinateScheme=ISO  VehLightsControl=off  HeadlightColor=[ 1, 1, 1 ]  HighBeamIntensity=100000  LowBeamIntensity=60000  HighBeamConeAngle=70  LowBeamConeAngle=70  LeftHeadlightOrientation=[ 0, 0 ]  RightHeadlightOrientation=[ 0, 0 ]  BrakelightIntensity=500  ReverselightIntensity=500  SignallightIntensity=500  SignallightPeriod=1  SignalPulseWidth=50  TransformOutportEnabled=off
      settings: LibrarySourceBlock=drivingsim3d/Simulation 3D Vehicle with Ground Following
  X1 : Constant  Value=info.SpotLocations(1,1)
  X10 : Constant  Value=info.SpotLocations(10,1)
  X11 : Constant  Value=info.SpotLocations(11,1)
  X12 : Constant  Value=info.SpotLocations(12,1)
  X13 : Constant  Value=info.SpotLocations(13,1)
  X14 : Constant  Value=info.SpotLocations(14,1)
  X15 : Constant  Value=info.SpotLocations(15,1)
  X16 : Constant  Value=info.SpotLocations(16,1)
  X17 : Constant  Value=info.SpotLocations(17,1)
  X18 : Constant  Value=info.SpotLocations(18,1)
  X19 : Constant  Value=info.SpotLocations(19,1)
  X2 : Constant  Value=info.SpotLocations(2,1)
  X20 : Constant  Value=info.SpotLocations(20,1)
  X21 : Constant  Value=info.SpotLocations(21,1)
  X22 : Constant  Value=info.SpotLocations(22,1)
  X23 : Constant  Value=info.SpotLocations(23,1)
  X3 : Constant  Value=info.SpotLocations(3,1)
  X4 : Constant  Value=info.SpotLocations(4,1)
  X5 : Constant  Value=info.SpotLocations(5,1)
  X6 : Constant  Value=16
  X7 : Constant  Value=info.SpotLocations(7,1)
  X9 : Constant  Value=info.SpotLocations(9,1)
  Y1 : Constant  Value=info.SpotLocations(1,2)
  Y10 : Constant  Value=info.SpotLocations(10,2)
  Y11 : Constant  Value=info.SpotLocations(11,2)
  Y12 : Constant  Value=info.SpotLocations(12,2)
  Y13 : Constant  Value=info.SpotLocations(13,2)
  Y14 : Constant  Value=info.SpotLocations(14,2)
  Y15 : Constant  Value=info.SpotLocations(15,2)
  Y16 : Constant  Value=info.SpotLocations(16,2)
  Y17 : Constant  Value=info.SpotLocations(17,2)
  Y18 : Constant  Value=info.SpotLocations(18,2)
  Y19 : Constant  Value=info.SpotLocations(19,2)
  Y2 : Constant  Value=info.SpotLocations(2,2)
  Y20 : Constant  Value=info.SpotLocations(20,2)
  Y21 : Constant  Value=info.SpotLocations(21,2)
  Y22 : Constant  Value=info.SpotLocations(22,2)
  Y23 : Constant  Value=info.SpotLocations(23,2)
  Y3 : Constant  Value=info.SpotLocations(3,2)
  Y4 : Constant  Value=info.SpotLocations(4,2)
  Y5 : Constant  Value=info.SpotLocations(5,2)
  Y6 : Constant  Value=17
  Y7 : Constant  Value=info.SpotLocations(7,2)
  Y9 : Constant  Value=info.SpotLocations(9,2)
  theta{1..7,9..23} (22 alike) : Constant  Value=-pi/2
  wires:
  Y15/1 -> Vehicle 15/2
  X15/1 -> Vehicle 15/1
  theta15/1 -> Radians to Degrees2/1
  X19/1 -> Vehicle 19/1
  Y19/1 -> Vehicle 19/2
  theta19/1 -> Radians to Degrees1/1
  Radians to Degrees2/1 -> Vehicle 15/3
  Radians to Degrees1/1 -> Vehicle 19/3
  Radians to Degrees3/1 -> Vehicle 16/3
  theta16/1 -> Radians to Degrees3/1
  X16/1 -> Vehicle 16/1
  Y16/1 -> Vehicle 16/2
  Y17/1 -> Vehicle 17/2
  X17/1 -> Vehicle 17/1
  theta17/1 -> Radians to Degrees4/1
  Radians to Degrees4/1 -> Vehicle 17/3
  Radians to Degrees6/1 -> Vehicle 20/3
  theta20/1 -> Radians to Degrees6/1
  X20/1 -> Vehicle 20/1
  Y20/1 -> Vehicle 20/2
  Radians to Degrees5/1 -> Vehicle 21/3
  theta21/1 -> Radians to Degrees5/1
  Y21/1 -> Vehicle 21/2
  X21/1 -> Vehicle 21/1
  X9/1 -> Vehicle 9/1
  Y9/1 -> Vehicle 9/2
  theta9/1 -> Radians to Degrees12/1
  Radians to Degrees12/1 -> Vehicle 9/3
  Radians to Degrees7/1 -> Vehicle 10/3
  theta13/1 -> Radians to Degrees8/1
  Y10/1 -> Vehicle 10/2
  theta12/1 -> Radians to Degrees9/1
  X10/1 -> Vehicle 10/1
  X13/1 -> Vehicle 13/1
  Y13/1 -> Vehicle 13/2
  theta10/1 -> Radians to Degrees7/1
  Y12/1 -> Vehicle 12/2
  Radians to Degrees8/1 -> Vehicle 13/3
  X11/1 -> Vehicle 11/1
  X12/1 -> Vehicle 12/1
  Radians to Degrees10/1 -> Vehicle 11/3
  theta11/1 -> Radians to Degrees10/1
  Y11/1 -> Vehicle 11/2
  Radians to Degrees9/1 -> Vehicle 12/3
  Radians to Degrees14/1 -> Vehicle 7/3
  theta7/1 -> Radians to Degrees14/1
  Y7/1 -> Vehicle 7/2
  X7/1 -> Vehicle 7/1
  X14/1 -> Vehicle 14/1
  Y14/1 -> Vehicle 14/2
  Radians to Degrees13/1 -> Vehicle 14/3
  theta14/1 -> Radians to Degrees13/1
  X2/1 -> Vehicle 2/1
  Y3/1 -> Vehicle 3/2
  Radians to Degrees16/1 -> Vehicle 3/3
  Y5/1 -> Vehicle 5/2
  theta6/1 -> Radians to Degrees15/1
  Y2/1 -> Vehicle 2/2
  Radians to Degrees15/1 -> Vehicle 6/3
  theta5/1 -> Radians to Degrees19/1
  Y4/1 -> Vehicle 4/2
  Y6/1 -> Vehicle 6/2
  theta4/1 -> Radians to Degrees17/1
  X3/1 -> Vehicle 3/1
  Radians to Degrees18/1 -> Vehicle 2/3
  Radians to Degrees19/1 -> Vehicle 5/3
  Radians to Degrees17/1 -> Vehicle 4/3
  theta2/1 -> Radians to Degrees18/1
  X6/1 -> Vehicle 6/1
  X5/1 -> Vehicle 5/1
  X4/1 -> Vehicle 4/1
  theta3/1 -> Radians to Degrees16/1
  Y23/1 -> Vehicle 23/2
  theta23/1 -> Radians to Degrees20/1
  Radians to Degrees20/1 -> Vehicle 23/3
  X22/1 -> Vehicle 22/1
  theta22/1 -> Radians to Degrees21/1
  X23/1 -> Vehicle 23/1
  Y22/1 -> Vehicle 22/2
  Radians to Degrees21/1 -> Vehicle 22/3
  theta18/1 -> Radians to Degrees22/1
  Radians to Degrees22/1 -> Vehicle 18/3
  Y18/1 -> Vehicle 18/2
  X18/1 -> Vehicle 18/1
  X1/1 -> Vehicle 1/1
  Y1/1 -> Vehicle 1/2
  Radians to Degrees11/1 -> Vehicle 1/3
  theta1/1 -> Radians to Degrees11/1

== system rlAutoParkingValet3D/Vehicle Dynamics and Sensing/Vehicle Mode Selector/Hold ==
  u : Inport
  Add : Sum
  Data Type Conversion : DataTypeConversion  OutDataTypeStr=boolean  SaturateOnIntegerOverflow=off  RndMeth=Floor
  Data Type Conversion2 : DataTypeConversion  OutDataTypeStr=double  SaturateOnIntegerOverflow=off  RndMeth=Floor
  Memory : Memory
  Saturation : Saturate  UpperLimit=1  LowerLimit=0
  y : Outport
  wires:
  u/1 -> Data Type Conversion2/1
  Add/1 -> Saturation/1, Memory/1
  Memory/1 -> Add/2
  Saturation/1 -> Data Type Conversion/1
  Data Type Conversion/1 -> y/1
  Data Type Conversion2/1 -> Add/1

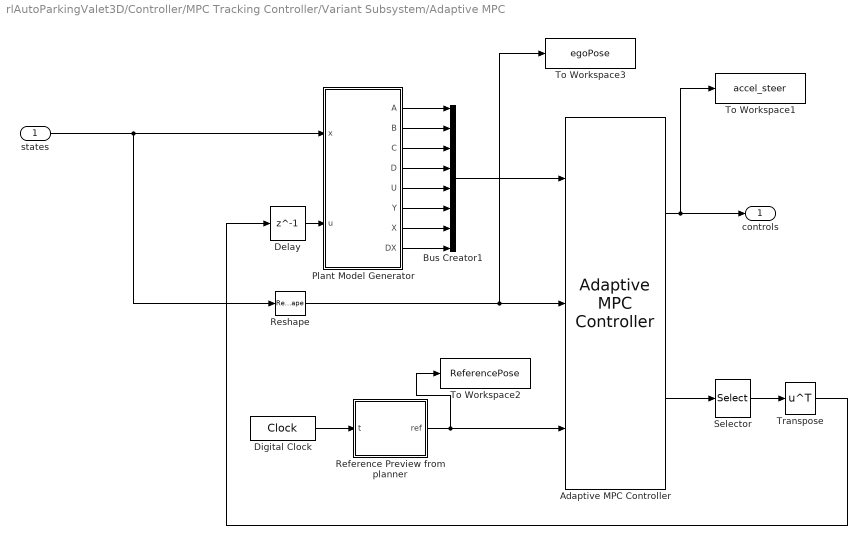
== system rlAutoParkingValet3D/Controller/MPC Tracking Controller/Variant Subsystem/Adaptive MPC ==
  states : Inport
  Adaptive MPC Controller : mpclib/Adaptive MPC Controller  SCDEnableBlockLinearizationSpecification=on  mpcobj=mpcobj  enable_value=0  updateMPCinCallerWorkspace=on  md_inport=off  mv_inport=off  uref_inport=off  return_cost=off  return_mvseq=on  return_qpstatus=off  return_xseq=off  return_state=off  return_ovseq=off  state_inport=on  isltv_plant=off  umin_inport=off  umax_inport=off  ymin_inport=off  ymax_inport=off  cc_inport=off  ywt_inport=off  uwt_inport=off  duwt_inport=off  rhoeps_inport=off  pm_inport=off  MaximumP=10  HorizonChoice=FixedHorizon  BlockDataType=double  SampleTimeInherited=off  switch_inport=off
  Bus Creator1 : BusCreator  Inputs=8
  Delay : Delay  DelayLength=1
  Digital Clock : DigitalClock  SampleTime=Ts
  Plant Model Generator : MATLAB Function  TreatAsAtomicUnit=on
  Reference Preview from planner : MATLAB Function  TreatAsAtomicUnit=on
  Reshape : Reshape  OutputDimensionality=Customize  OutputDimensions=[3,1]
  Selector : Selector  NumberOfDimensions=2  InputPortWidth=3  IndexOptions=Index vector (dialog),Select all  Indices=2,2  OutputSizes=1,1
  To Workspace1 : ToWorkspace  VariableName=accel_steer  SaveFormat=Timeseries  SampleTime=-1
  To Workspace2 : ToWorkspace  VariableName=ReferencePose  SaveFormat=Timeseries  SampleTime=-1
  To Workspace3 : ToWorkspace  VariableName=egoPose  SaveFormat=Timeseries  SampleTime=-1
  Transpose : Math  Operator=transpose  SignedPower=on
  controls : Outport
  wires:
  Adaptive MPC Controller/1 -> controls/1, To Workspace1/1
  Selector/1 -> Transpose/1
  Delay/1 -> Plant Model Generator/2(u)
  Reshape/1 -> To Workspace3/1, Adaptive MPC Controller/2
  Plant Model Generator/1(A) -> Bus Creator1/1
  Plant Model Generator/6(Y) -> Bus Creator1/6
  Transpose/1 -> Delay/1
  Plant Model Generator/3(C) -> Bus Creator1/3
  states/1 -> Reshape/1, Plant Model Generator/1(x)
  Plant Model Generator/8(DX) -> Bus Creator1/8
  Reference Preview from planner/1(ref) -> To Workspace2/1, Adaptive MPC Controller/3
  Plant Model Generator/2(B) -> Bus Creator1/2
  Plant Model Generator/5(U) -> Bus Creator1/5
  Adaptive MPC Controller/2 -> Selector/1
  Plant Model Generator/4(D) -> Bus Creator1/4
  Plant Model Generator/7(X) -> Bus Creator1/7
  Digital Clock/1 -> Reference Preview from planner/1(t)
  Bus Creator1/1 -> Adaptive MPC Controller/1

== system rlAutoParkingValet3D/Controller/MPC Tracking Controller/Variant Subsystem/LQR ==
  states : Inport
  Digital Clock1 : DigitalClock  SampleTime=Ts
  K_lqr : Constant  Value=K_lqr
  MATLAB Function : MATLAB Function  TreatAsAtomicUnit=on
  Reference Preview from planner : MATLAB Function  TreatAsAtomicUnit=on
  Reshape1 : Reshape  OutputDimensionality=Customize  OutputDimensions=[3,1]
  To Workspace : ToWorkspace  VariableName=egoPose  SaveFormat=Timeseries  SampleTime=-1
  To Workspace1 : ToWorkspace  VariableName=accel_steer  SaveFormat=Timeseries  SampleTime=-1
  To Workspace2 : ToWorkspace  VariableName=ReferencePose  SaveFormat=Timeseries  SampleTime=-1
  controls : Outport
  wires:
  Reference Preview from planner/1(ref) -> MATLAB Function/2(ReferencePose), To Workspace2/1
  Reshape1/1 -> To Workspace/1, MATLAB Function/1(egoPose)
  states/1 -> Reshape1/1
  K_lqr/1 -> MATLAB Function/3(K_lqr)
  MATLAB Function/1(accel_steer) -> To Workspace1/1, controls/1
  Digital Clock1/1 -> Reference Preview from planner/1(t)
